simulink model "model_validation_lab"  (R2022b)
settings: Solver=VariableStepAuto  StartTime=0.0  StopTime=10.0  RelTol=1e-3
undefined symbols (not defined in the file or in its folder): A, B, C, Continuous, D, g0, Ip, Ir, k, La, Lp, Lr, mp, mr, phi_dot_init, phi_init, R_tilde, Ra, rot_pend, theta_dot_init, theta_init, Time
libraries: simulink_extras x4, ctrlSharedLib x1
settings Model: Creator=Mark  LastModifiedBy=Mark
settings OptimizationCC: ReuseModelBlockBuffer=on

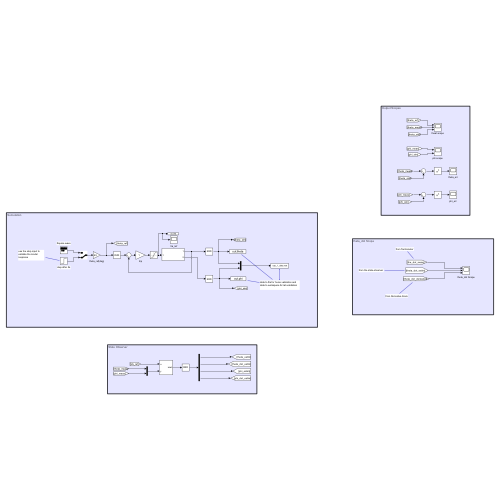
[thumbnail: Simulink's stored preview of the top-level diagram]
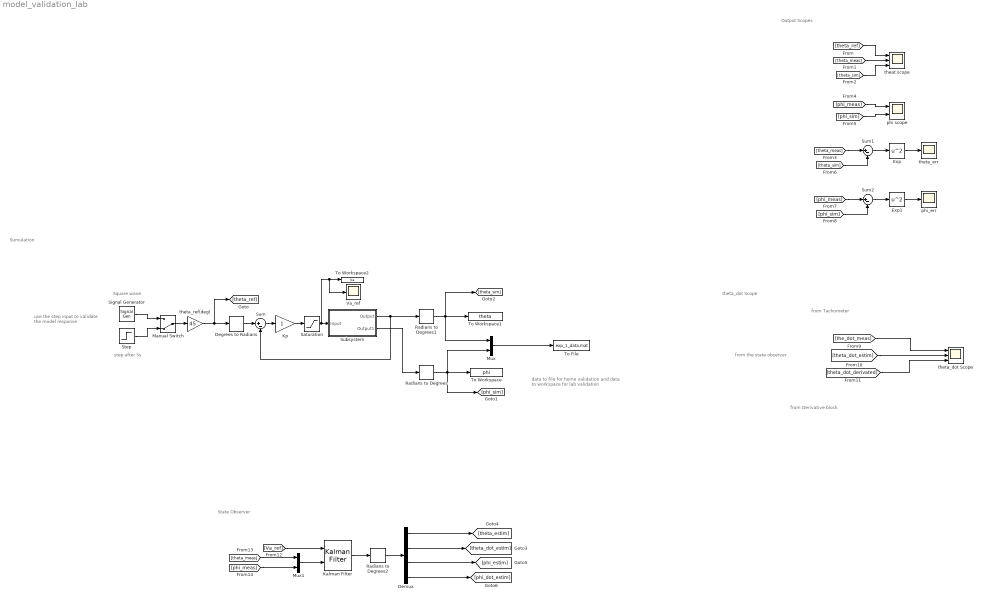
== system model_validation_lab ==
  note: State Observer
  note: Sumulation
  note: theta_dot Scope
  note: from Tachometer
  note: from Derivative block
  note: from the state observer
  note: Output Scopes
  note: use the step input to validate the model response
  note: data to file for home validation and data to workspace for lab validation
  note: step after 5s
  note: Square wave
  Degrees to Radians : simulink_extras/Transformations/Degrees to Radians
  Demux : Demux
  Exp : Math  Operator=square
  Exp1 : Math  Operator=square
  Kalman Filter : ctrlSharedLib/Kalman Filter  TimeDomain=Continuous-Time  UseCurrentEstimator=on  ModelSource=Individual A, B, C, D matrices  ModelSourceVariable=ss(0.95,1,1,0,1)  A=A  B=B  C=C  D=D  NumberOfStates=1  NumberOfInputs=1  NumberOfOutputs=1  InitialEstimateSource=Dialog  X0=0  P0=10  UseK=off  UseGH=off  NumberOfProcessNoiseInputs=1  G=1  TimeInvariantG=on  H=0  TimeInvariantH=on  Q=Q_tilde  TimeInvariantQ=on  R=R_tilde  TimeInvariantR=on  N=0  TimeInvariantN=on  AddInputPort=on  AddEnablePort=off  OutputEstimatedY=off  OutputP=off  Ts=-1
  Kp : Gain
  Manual Switch : ManualSwitch  CurrentSetting=0
  Mux : Mux  Inputs=2
  Mux1 : Mux  Inputs=2
  Radians to Degrees : simulink_extras/Transformations/Radians to Degrees
  Radians to Degrees1 : simulink_extras/Transformations/Radians to Degrees
  Radians to Degrees2 : simulink_extras/Transformations/Radians to Degrees
  Saturation : Saturate  UpperLimit=10  LowerLimit=-10
  Signal Generator : SignalGenerator  WaveForm=square  Frequency=0.05
  Step : Step  Time=5  SampleTime=0
  Subsystem : Subsystem
  Sum : Sum  Inputs=|+-
  Sum1 : Sum  Inputs=|+-
  Sum2 : Sum  Inputs=|+-
  To File : ToFile  Filename=exp_1_data.mat  MatrixName=angle
  To Workspace : ToWorkspace  VariableName=phi  SampleTime=-1
  To Workspace1 : ToWorkspace  VariableName=theta  SampleTime=-1
  To Workspace2 : ToWorkspace  VariableName=Va  SampleTime=-1
  Va_ref : Scope
  phi scope : Scope  NumInputPorts=2
  phi_err : Scope
  theat scope : Scope  NumInputPorts=3
  theta_dot Scope : Scope  NumInputPorts=3
  theta_err : Scope
  theta_ref(deg) : Gain  Gain=45
  wires:
  Mux/1 -> To File/1
  Kp/1 -> Saturation/1
  Saturation/1 -> Va_ref/1, To Workspace2/1, Subsystem/1(Input)
  Step/1 -> Manual Switch/2
  theta_ref(deg)/1 -> [theta_ref], Degrees to Radians/1
  Signal Generator/1 -> Manual Switch/1
  Radians to Degrees1/1 -> [theta_sim], To Workspace1/1, Mux/1
  Degrees to Radians/1 -> Sum/1
  Subsystem/2(Output1) -> Radians to Degrees/1
  Radians to Degrees/1 -> Mux/2, To Workspace/1, [phi_sim]
  Subsystem/1(Output) -> Radians to Degrees1/1, Sum/2
  Sum/1 -> Kp/1
  Manual Switch/1 -> theta_ref(deg)/1
  [theta_meas] -> theat scope/2
  [theta_sim] -> theat scope/3
  [theta_ref] -> theat scope/1
  [phi_meas] -> phi scope/1
  [phi_sim] -> phi scope/2
  Exp/1 -> theta_err/1
  Sum1/1 -> Exp/1
  [theta_meas] -> Sum1/1
  [theta_sim] -> Sum1/2
  [phi_sim] -> Sum2/2
  Exp1/1 -> phi_err/1
  Sum2/1 -> Exp1/1
  [phi_meas] -> Sum2/1
  [the_dot_meas] -> theta_dot Scope/1
  [theta_dot_estim] -> theta_dot Scope/2
  [theta_dot_derivated] -> theta_dot Scope/3
  Radians to Degrees2/1 -> Demux/1
  Kalman Filter/1 -> Radians to Degrees2/1
  Mux1/1 -> Kalman Filter/2
  [Va_ref] -> Kalman Filter/1
  [theta_meas] -> Mux1/1
  [phi_meas] -> Mux1/2
  Demux/2 -> [theta_dot_estim]
  Demux/1 -> [theta_estim]
  Demux/3 -> [phi_estim]
  Demux/4 -> [phi_dot_estim]

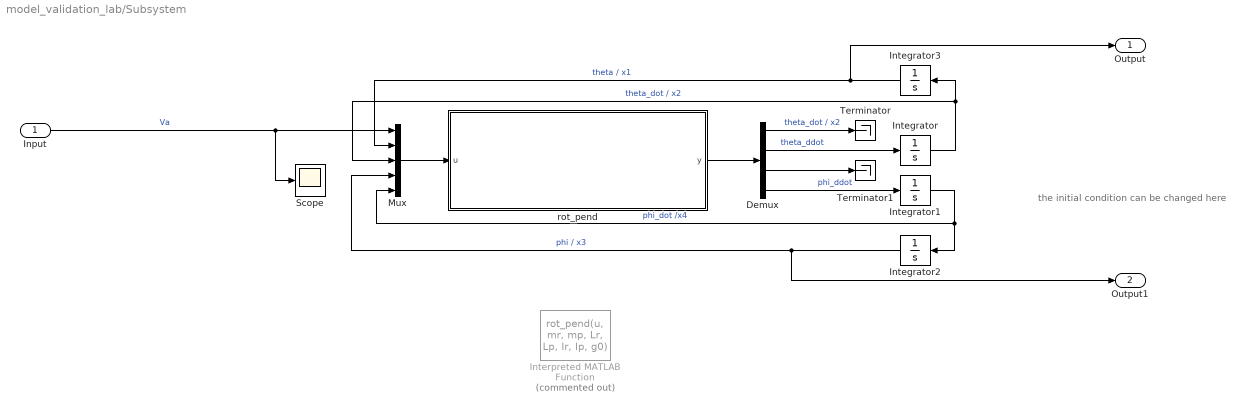
== system model_validation_lab/Subsystem ==
  note: the initial condition can be changed here
  Input : Inport
  Demux : Demux
  Integrator : Integrator  InitialCondition=theta_dot_init
  Integrator1 : Integrator  InitialCondition=phi_dot_init
  Integrator2 : Integrator  InitialCondition=phi_init
  Integrator3 : Integrator  InitialCondition=theta_init
  Interpreted MATLAB Function : MATLABFcn  Commented=on  MATLABFcn=rot_pend(u, mr, mp, Lr, Lp, Ir, Ip, g0)  OutputDimensions=4  OutputSignalType=real
  Mux : Mux  Inputs=5
  Scope : Scope
  Terminator : Terminator
  Terminator1 : Terminator
  rot_pend : Subsystem
  Output : Outport
  Output1 : Outport  Port=2
  wires:
  Input/1 -> Scope/1, Mux/1  "Va"
  Integrator2/1 -> Output1/1, Mux/4  "phi / x3"
  Integrator/1 -> Integrator3/1, Mux/3  "theta_dot / x2"
  Mux/1 -> rot_pend/1(u)
  rot_pend/1(y) -> Demux/1
  Integrator1/1 -> Mux/5, Integrator2/1  "phi_dot /x4"
  Integrator3/1 -> Mux/2, Output/1  "theta / x1"
  Demux/4 -> Integrator1/1  "phi_ddot"
  Demux/2 -> Integrator/1  "theta_ddot"
  Demux/1 -> Terminator/1  "theta_dot / x2"
  Demux/3 -> Terminator1/1

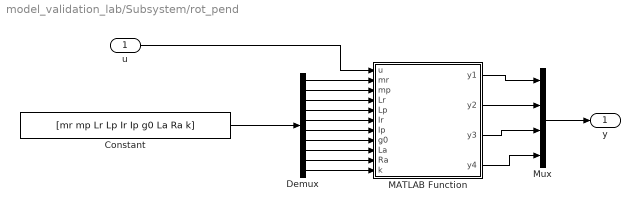
== system model_validation_lab/Subsystem/rot_pend ==
  u : Inport
  Constant : Constant  Value=[mr mp Lr Lp Ir Ip g0 La Ra k]  VectorParams1D=off
  Demux : Demux  Outputs=10
  MATLAB Function : MATLAB Function  TreatAsAtomicUnit=on
  Mux : Mux
  y : Outport
  wires:
  Demux/3 -> MATLAB Function/4(Lr)
  Demux/5 -> MATLAB Function/6(Ir)
  Demux/4 -> MATLAB Function/5(Lp)
  Demux/7 -> MATLAB Function/8(g0)
  Demux/2 -> MATLAB Function/3(mp)
  Demux/6 -> MATLAB Function/7(Ip)
  Demux/1 -> MATLAB Function/2(mr)
  u/1 -> MATLAB Function/1(u)
  Constant/1 -> Demux/1
  MATLAB Function/1(y1) -> Mux/1
  MATLAB Function/2(y2) -> Mux/2
  MATLAB Function/3(y3) -> Mux/3
  MATLAB Function/4(y4) -> Mux/4
  Mux/1 -> y/1
  Demux/8 -> MATLAB Function/9(La)
  Demux/9 -> MATLAB Function/10(Ra)
  Demux/10 -> MATLAB Function/11(k)

== matlab function model_validation_lab/Subsystem/rot_pend/MATLAB Function ==
  data: u input; y1 output; mr input; mp input; Lr input; Lp input; Ir input; Ip input; g0 input; La input; Ra input; y2 output; y3 output; y4 output; k input
function [y1,y2,y3,y4] = rot_pend(u, mr, mp, Lr, Lp, Ir, Ip, g0,La, Ra, k)
%UNTITLED Summary of this function goes here
%   Detailed explanation goes here
% u(1) = Va
x1 = u(2) ; % theta
x2 = u(3) ; % theta_dot
x3 = u(4) ; % phi
x4 = u(5) ; % phi_dot

H = [(mp*(Lr^2+(Lp^2*(sin(x3))^2)))+Ir           mp*Lr*Lp*cos(x3);
                     mp*Lr*Lp*cos(x3)                              (mp*Lp^2)+Ip] ;

Q = [mp*Lp^2*sin(x3)*cos(x3)*x4                     (mp*Lp^2*sin(x3)*cos(x3)*x2)-(mp*Lr*Lp*sin(x3)*x4);
     -mp*Lp^2*sin(x3)*cos(x3)*x4                                                   0                                   ] ;

g = [           0     ;
     -mp*g0*Lp*sin(x3)] ;
tau = [((k/Ra)*u(1))-((k^2/Ra)*x2);
                    0                   ] ;

q_ddot = H\[tau - Q*[x2 x4]' - g] ;


y1 = x2 ;
y2 = q_ddot(1) ;
y3 = x4 ;
y4 = q_ddot(2) ;


%Ir+mr*(Lr/2)^2)
